simulink model "engduino_drivers"  (R2015a)
settings: Solver=ode45  StartTime=0.0  StopTime=10.0  RelTol=1e-3
settings Model: CovSFcnEnable=off  Creator=Cosmin  LastModifiedBy=kkhoo
settings OptimizationCC: OptimizeModelRefInitCode=on  LifeSpan=1
settings DebuggingCC: UnderspecifiedInitializationDetection=Classic  MergeDetectMultiDrivingBlocksExec=none  StrictBusMsg=Warning
settings HardwareCC: ProdBitPerInt=16  ProdBitPerPointer=8  ProdIntDivRoundTo=Zero  ProdEndianess=LittleEndian  ProdWordSize=8  ProdHWDeviceType=Atmel->AVR
settings RTWCC: SystemTargetFile=realtime.tlc  GenerateMakefile=off  TemplateMakefile=realtime.tmf  Description=Run on Target Hardware  RTWVerbose=off  CustomSource=src/Engduino.h src/engduino_wrappers.cpp
settings CodeAppCC: IgnoreCustomStorageClasses=off
settings STFCustomTargetCC: CombineOutputUpdateFcns=on  SupportContinuousTime=off  SupportVariableSizeSignals=off
settings ERTTargetCC: SupportContinuousTime=off  SupportVariableSizeSignals=off  ERTCustomFileTemplate=realtime_file_process.tlc

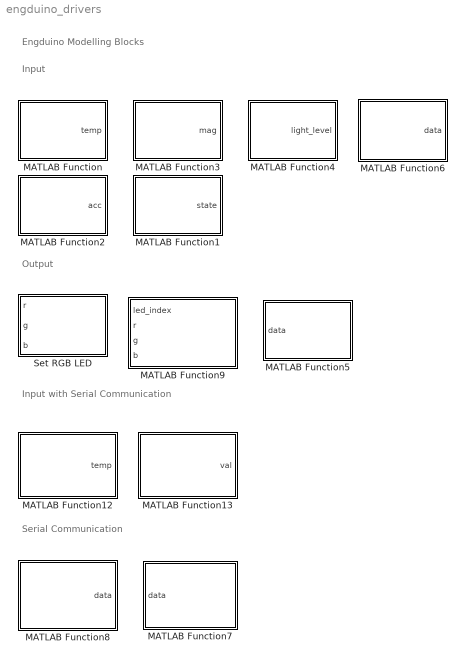
== system engduino_drivers ==
  note: Input
  note: Engduino Modelling Blocks
  note: Output
  note: Input with Serial Communication
  note: Serial Communication
  MATLAB Function : MATLAB Function  LoadFcn=|  TreatAsAtomicUnit=on  mask(Thermistor){}
      | set_param(gcs, 'CustomSource', strjoin(unique([strsplit(get_param(gcs, 'CustomSource')) ...
      |  'src/engduino_wrappers.cpp' 'src/Engduino.h'])));
      mask help: Outputs the temperature in milli degrees celsius.
  MATLAB Function1 : MATLAB Function  LoadFcn=|  TreatAsAtomicUnit=on  mask(Button){}
      | set_param(gcs, 'CustomSource', strjoin(unique([strsplit(get_param(gcs, 'CustomSource')) ...
      |  'src/engduino_wrappers.cpp' 'src/Engduino.h'])));
      mask help: Outputs 1 if the button is pressed, 0 otherwise.
  MATLAB Function12 : MATLAB Function  LoadFcn=|  TreatAsAtomicUnit=on  mask(Thermistor){}
      | set_param(gcs, 'CustomSource', strjoin(unique([strsplit(get_param(gcs, 'CustomSource')) ...
      |  'src/engduino_wrappers.cpp' 'src/Engduino.h'])));
      mask help:
      | Send the data in millis degree celsius via serial communication,
      | Outputs the temperature in milli degrees celsius,
      | Data output type is uint16_t
  MATLAB Function13 : MATLAB Function  LoadFcn=|  TreatAsAtomicUnit=on  mask(Photodiode){}
      | set_param(gcs, 'CustomSource', strjoin(unique([strsplit(get_param(gcs, 'CustomSource')) ...
      |  'src/engduino_wrappers.cpp' 'src/Engduino.h'])));
      mask help:
      | Send the light intensity data in the range between 0-1023 via serial communication,
      | Outputs the light intensity data in the range between 0-1023
      | Data output type is uint16_t
  MATLAB Function2 : MATLAB Function  LoadFcn=|  TreatAsAtomicUnit=on  mask(Accelerometer
Accelerometer){}
      | set_param(gcs, 'CustomSource', strjoin(unique([strsplit(get_param(gcs, 'CustomSource')) ...
      |  'src/engduino_wrappers.cpp' 'src/Engduino.h'])));
      mask help: Outputs a three components of the acceleration filed as a [x y z] vector.
  MATLAB Function3 : MATLAB Function  LoadFcn=|  TreatAsAtomicUnit=on  mask(Magnetometer){}
      | set_param(gcs, 'CustomSource', strjoin(unique([strsplit(get_param(gcs, 'CustomSource')) ...
      |  'src/engduino_wrappers.cpp' 'src/Engduino.h'])));
      mask help: Outputs a three components of the magnetic filed as a [x y z] vector.
  MATLAB Function4 : MATLAB Function  LoadFcn=|  TreatAsAtomicUnit=on  mask(Photodiode){}
      | set_param(gcs, 'CustomSource', strjoin(unique([strsplit(get_param(gcs, 'CustomSource')) ...
      |  'src/engduino_wrappers.cpp' 'src/Engduino.h'])));
      mask help: Outputs the light level as a uint16, in the range 0-1023.
  MATLAB Function5 : MATLAB Function  LoadFcn=|  TreatAsAtomicUnit=on  mask(IR Send){}
      | set_param(gcs, 'CustomSource', strjoin(unique([strsplit(get_param(gcs, 'CustomSource')) ...
      |  'src/engduino_wrappers.cpp' 'src/Engduino.h'])));
      mask help: Sends one byte at a time using the infrared transmitter.
  MATLAB Function6 : MATLAB Function  LoadFcn=|  TreatAsAtomicUnit=on  mask(IR Receive){}
      | set_param(gcs, 'CustomSource', strjoin(unique([strsplit(get_param(gcs, 'CustomSource')) ...
      |  'src/engduino_wrappers.cpp' 'src/Engduino.h'])));
      mask help: Receives one byte at a time using the infrared transmitter.
  MATLAB Function7 : MATLAB Function  LoadFcn=|  TreatAsAtomicUnit=on  mask(Serial Transmission){}
      | set_param(gcs, 'CustomSource', strjoin(unique([strsplit(get_param(gcs, 'CustomSource')) ...
      |  'src/engduino_wrappers.cpp' 'src/Engduino.h'])));
      mask help: Receive data in double and send it via Serial Communication. The data is sent in their String representation.
  MATLAB Function8 : MATLAB Function  LoadFcn=|  TreatAsAtomicUnit=on  mask(Serial Transmission){}
      | set_param(gcs, 'CustomSource', strjoin(unique([strsplit(get_param(gcs, 'CustomSource')) ...
      |  'src/engduino_wrappers.cpp' 'src/Engduino.h'])));
      mask help:
      | Read the data sent to Engduino via serial communication and output the data as uint16_t data type.
      | Output 0 if no data is received.
      | Implementation: Serial data is received in their ASCII DEC value. You may use it to control the Engduino to do something.
  MATLAB Function9 : MATLAB Function  LoadFcn=|  TreatAsAtomicUnit=on  mask(RGB LED){}
      | set_param(gcs, 'CustomSource', strjoin(unique([strsplit(get_param(gcs, 'CustomSource')) ...
      |  'src/engduino_wrappers.cpp' 'src/Engduino.h'])));
      mask help:
      | Control the Red, Green and Blue color values of the LED specified by the LED index values.
      | Both the LED index and the three color values are of type uint8 and must be in the range 0-15.
  Set RGB LED : MATLAB Function  LoadFcn=|  TreatAsAtomicUnit=on  mask(RGB LED){led_index=0}
      | set_param(gcs, 'CustomSource', strjoin(unique([strsplit(get_param(gcs, 'CustomSource')) ...
      |  'src/engduino_wrappers.cpp' 'src/Engduino.h'])));
      mask prompts: led_index "LED index"
      mask help:
      | Control the Red, Green and Blue color values of the LED specified by the LED index parameter.
      | Both the LED index and the three color values are of type uint8 and must be in the range 0-15.
      settings: AttributesFormatString=LED %<led_index>

== matlab function engduino_drivers/MATLAB Function1 ==
  data: state output
function state = button()

state = 0;

if strcmp(coder.target, 'rtw')
    state = coder.ceval('button_wrapper');
end

== matlab function engduino_drivers/MATLAB Function ==
  data: temp output
function temp = thermistor()

temp = 0.0;

if strcmp(coder.target, 'rtw')
    temp = coder.ceval('thermistor_wrapper');
end

== matlab function engduino_drivers/Set RGB LED ==
  data: led_index parameter uint8 [0..15]; r input uint8 [0..15]; g input uint8 [0..15]; b input uint8 [0..15]
function rgb_led(led_index, r, g, b)

if strcmp(coder.target, 'rtw')
    coder.ceval('rgb_leds_wrapper', led_index, r, g, b);
end

== matlab function engduino_drivers/MATLAB Function7 ==
  data: data input
function serial_print(data)

if strcmp(coder.target, 'rtw')
    coder.ceval('print_data_serial_wrapper', data);
end

== matlab function engduino_drivers/MATLAB Function2 ==
  data: acc output size=[1, 3]
function acc = accelerometer()

acc = [0.0 0.0 0.0];

if strcmp(coder.target, 'rtw')
    coder.ceval('accelerometer_wrapper', coder.ref(acc));
end

== matlab function engduino_drivers/MATLAB Function8 ==
  data: data output
function data = read_serial()

data = 0;

if strcmp(coder.target, 'rtw')
    data = coder.ceval('read_data_serial_wrapper');
end

== matlab function engduino_drivers/MATLAB Function9 ==
  data: led_index input; r input; g input; b input
function rgb_led_selector( led_index,r, g, b)

if strcmp(coder.target, 'rtw')
    coder.ceval('rgb_leds_wrapper', led_index, r, g, b);
end

== matlab function engduino_drivers/MATLAB Function3 ==
  data: mag output size=[1, 3]
function mag = magnetometer()

mag = [0.0 0.0 0.0];

if strcmp(coder.target, 'rtw')
    coder.ceval('magnetometer_wrapper', coder.ref(mag));
end

== matlab function engduino_drivers/MATLAB Function12 ==
  data: temp output
function temp = thermistor_serial()
temp = 0.0;
if strcmp(coder.target, 'rtw')
    temp=coder.ceval('read_thermistor_wrapper');
end

== matlab function engduino_drivers/MATLAB Function13 ==
  data: val output
function val = photodiode_serial()
val = 0;
if strcmp(coder.target, 'rtw')
    val = coder.ceval('read_photodiode_wrapper');
end

== matlab function engduino_drivers/MATLAB Function4 ==
  data: light_level output
function light_level = photodiode()

light_level = 0.0;

if strcmp(coder.target, 'rtw')
    light_level = coder.ceval('photodiode_wrapper');
end

== matlab function engduino_drivers/MATLAB Function5 ==
  data: data input uint8
function ir_send(data)

if strcmp(coder.target, 'rtw')
    coder.ceval('ir_send_wrapper', data);
end

== matlab function engduino_drivers/MATLAB Function6 ==
  data: data output uint8
function data = ir_receive()

data = uint8(0);

if strcmp(coder.target, 'rtw')
    data = coder.ceval('ir_receive_wrapper');
end
